simulink model "mcb_bldc_sixstep_f28069mLaunchPad"  (R2023b)
settings: Solver=FixedStepDiscrete  StartTime=0.0  StopTime=2  RelTol=1e-3  EnableMultiTasking=on
InitFcn:
  | mcb_bldc_sixstep_f28069mLaunchPad_data;
values from neighbouring files (symbols this model uses):
  bldc = mcb_SetPMSMMotorParameters('D60MR6430')    [mcb_bldc_sixstep_f28069mLaunchPad_data.m]
  inverter = mcb_SetInverterParameters('SBLMB500')    [mcb_bldc_sixstep_f28069mLaunchPad_data.m]
  PI_params = mcb_SetControllerParameters(bldc,inverter,PU_System,T_pwm,2*Ts,Ts_speed)    [mcb_bldc_sixstep_f28069mLaunchPad_data.m]
  PWM_frequency = 20e3    (= 20000)    [mcb_bldc_sixstep_f28069mLaunchPad_data.m]
  target = mcb_SetProcessorDetails('F28069M',PWM_frequency)    [mcb_bldc_sixstep_f28069mLaunchPad_data.m]
  Ts = 0.03    [dataMonitoringArr.m]    (also in mcb_bldc_sixstep_f28069mLaunchPad_data.m = 5e-05)
  Ts_motor = T_pwm/2    (= 2.5e-05)    [mcb_bldc_sixstep_f28069mLaunchPad_data.m]
  Ts_motor_simscape = T_pwm/100    (= 5e-07)    [mcb_bldc_sixstep_f28069mLaunchPad_data.m]
  Ts_simulink = T_pwm/2    (= 2.5e-05)    [mcb_bldc_sixstep_f28069mLaunchPad_data.m]
  Ts_speed = 10*Ts    (= 0.0005)    [mcb_bldc_sixstep_f28069mLaunchPad_data.m]
undefined symbols (not defined in the file or in its folder): Down, GPTRIP1SEL, GPTRIP2SEL, TZ1, TZ2, Up
libraries: nesl_utility x14, simulink x9, fl_lib x9, c2802xlib x7, mcbcontrolslib x6, c280xlib x6, mcbpositiondecoderlib x5, c2806xlib x5, ee_lib x5, slpidlib x2, svdschedulerlib x2
(part 1 of 3)
settings Model: SILPILSystemUnderTest=refmodels  ExtModeTrigDuration=8  VariantFading=off  Creator=The MathWorks, Inc.  LastModifiedBy=Tefilus
settings SolverCC: AlgebraicLoopSolver=TrustRegion  AutoInsertRateTranBlk=on
settings DataIOCC: LimitDataPoints=on  SaveFormat=Array  SaveOutput=off  SaveTime=off  ReturnWorkspaceOutputs=off
settings OptimizationCC: DefaultParameterBehavior=Inlined  DefaultUnderspecifiedDataType=single  OptimizeBlockIOStorage=off  BufferReuse=off  ReuseModelBlockBuffer=off  GlobalBufferReuse=off  ExpressionFolding=off  ExpressionDepthLimit=2147483647  LocalBlockOutputs=off  InitFltsAndDblsToZero=on  NoFixptDivByZeroProtection=on  EfficientFloat2IntCast=on  EfficientMapNaN2IntZero=off  LifeSpan=inf  MaxStackSize=1024  OptimizeDataStoreBuffers=off  BusAssignmentInplaceUpdate=off  DenormalBehavior=FlushToZero  EfficientTunableParamExpr=on
settings DebuggingCC: AlgebraicLoopMsg=error  ArtificialAlgebraicLoopMsg=error  CheckSSInitialOutputMsg=off  MergeDetectMultiDrivingBlocksExec=none  SolverPrmCheckMsg=warning  InheritedTsInSrcMsg=none  MultiTaskDSMMsg=none  MultiTaskCondExecSysMsg=none  TasksWithSamePriorityMsg=none  SigSpecEnsureSampleTimeMsg=none  ParameterPrecisionLossMsg=none  ParameterTunabilityLossMsg=error  FcnCallInpInsideContextMsg=warning  UnconnectedInputMsg=warning  UnconnectedOutputMsg=warning  UnconnectedLineMsg=warning  AllowSymbolicDim=off  StateNameClashWarn=warning  SFUnexpectedBacktrackingDiag=warning  SFNoUnconditionalDefaultTransitionDiag=warning  SFExecutionAtInitializationDiag=none  ArithmeticOperatorsInVariantConditions=warning
settings HardwareCC: ProdBitPerChar=16  ProdBitPerInt=16  ProdBitPerPointer=32  ProdBitPerSizeT=32  ProdBitPerPtrDiffT=32  ProdLargestAtomicInteger=Integer  ProdLargestAtomicFloat=None  ProdWordSize=16  ProdLongLongMode=on  ProdHWDeviceType=Texas Instruments->C2000  TargetBitPerChar=16  TargetBitPerInt=16  TargetLargestAtomicInteger=Integer  TargetLongLongMode=on  TargetIntDivRoundTo=Zero  TargetEndianess=LittleEndian  TargetWordSize=16  TargetHWDeviceType=Texas Instruments->C2000  ProdEqTarget=off
settings ModelReferenceCC: EnableRefExpFcnMdlSchedulingChecks=on  PropagateSignalLabelsOutOfModel=off
settings SFSimCC: SimUseLocalCustomCode=off  MATLABDynamicMemAlloc=off
settings RTWCC: Description=Embedded Coder  SystemTargetFile=ert.tlc  HardwareBoard=TI Piccolo F28069M LaunchPad  TemplateMakefile=ert_default_tmf  PostCodeGenCommand=; codertarget.postCodeGenHookCommand(h)  GenerateReport=on  RTWUseLocalCustomCode=off  Toolchain=Texas Instruments Code Composer Studio (C2000)  IncludeHyperlinkInReport=on  GenerateTraceInfo=on  GenerateTraceReport=on  GenerateTraceReportSl=on  GenerateTraceReportSf=on  GenerateTraceReportEml=on  DLArmComputeVersion=19.05
settings CodeAppCC: IgnoreCustomStorageClasses=off  CustomSymbolStrType=$N$R$M  StateflowObjectComments=on  InternalIdentifier=Classic
settings ERTTargetCC: TargetFcnLib=ansi_tfl_tmw_new.mat  CodeReplacementLibrary=TI C28x  MultiwordLength=2048  ParMdlRefBuildCompliant=off  CompOptLevelCompliant=off  ConcurrentExecutionCompliant=off  CPPClassGenCompliant=off  ExtModeStaticAllocSize=2000  ExtModeMexFile=TIC2000ExternalModeOpen  ExtModeIntrfLevel=Level2 - Open  ConvertIfToSwitch=off  SuppressUnreachableDefaultCases=off  MemSecPackage=tic2000demospkg
settings ConfigComp: CovMetricSettings=dw  CovSaveCumulativeToWorkspaceVar=on  CovSaveSingleToWorkspaceVar=on  CovExternalEMLEnable=off  CovSFcnEnable=off

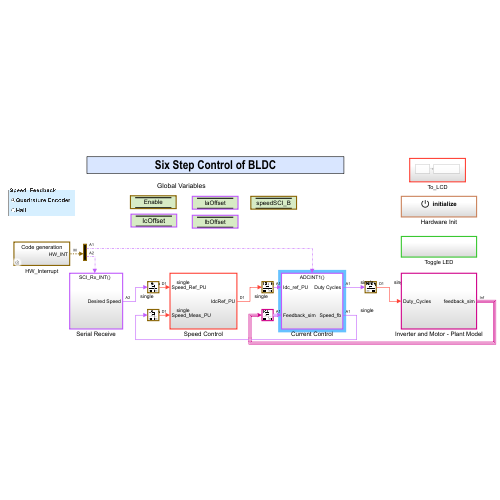
[thumbnail: Simulink's stored preview of the top-level diagram]
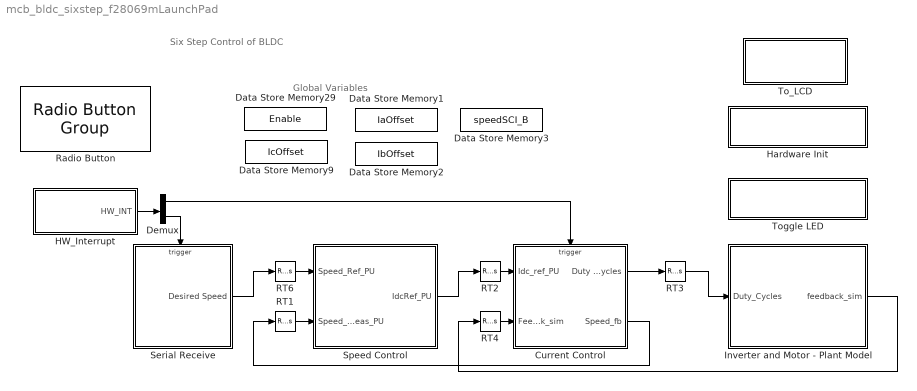
== system mcb_bldc_sixstep_f28069mLaunchPad ==
  note: Six Step Control of BLDC
  note: Global Variables
  Current Control : Subsystem
      settings: RTWSystemCode=Nonreusable function
  Data Store Memory1 : DataStoreMemory  DataStoreName=IaOffset  InitialValue=inverter.CtSensAOffset  ShowAdditionalParam=off
  Data Store Memory2 : DataStoreMemory  DataStoreName=IbOffset  InitialValue=inverter.CtSensBOffset  ShowAdditionalParam=off
  Data Store Memory29 : DataStoreMemory  DataStoreName=Enable  ShowAdditionalParam=off  OutDataTypeStr=boolean
  Data Store Memory3 : DataStoreMemory  DataStoreName=speedSCI_B  InitialValue=inverter.CtSensAOffset  ShowAdditionalParam=off
  Data Store Memory9 : DataStoreMemory  DataStoreName=IcOffset  InitialValue=inverter.CtSensBOffset  ShowAdditionalParam=off
  Demux : Demux  Outputs=2
  HW_Interrupt : Subsystem  Variant=on  VariantControlMode=sim codegen switching
  Hardware Init : Subsystem  TreatAsAtomicUnit=on
  Inverter and Motor - Plant Model : Subsystem
  RT1 : RateTransition  Deterministic=off  OutPortSampleTime=Ts_speed
  RT{2..4,6} (4 alike) : RateTransition  Deterministic=off
  Radio Button : RadioButtonGroup  LabelPosition=Hide  SelectedLabel=Quadrature Encoder  ButtonGroupName=Speed_Feedback
      settings: Values={{'Quadrature Encoder', 'Hall'}, [0 1]}
  Serial Receive : Subsystem  SystemSampleTime=1e-3
  Speed Control : Subsystem  TreatAsAtomicUnit=on  SystemSampleTime=Ts_speed
  To_LCD : Subsystem  TreatAsAtomicUnit=on  SystemSampleTime=Ts_speed
      settings: RTWFcnNameOpts=Use subsystem name  RTWFileNameOpts=Use subsystem name
  Toggle LED : Subsystem
  wires:
  RT3/1 -> Inverter and Motor - Plant Model/1(Duty_Cycles)
  Inverter and Motor - Plant Model/1(feedback_sim) -> RT4/1
  Demux/1 -> Current Control/Trigger
  RT6/1 -> Speed Control/1(Speed_Ref_PU)
  RT1/1 -> Speed Control/2(Speed_Meas_PU)
  Speed Control/1(IdcRef_PU) -> RT2/1
  Demux/2 -> Serial Receive/Trigger
  Current Control/1(Duty Cycles) -> RT3/1
  HW_Interrupt/1(HW_INT) -> Demux/1
  Current Control/2(Speed_fb) -> RT1/1
  RT4/1 -> Current Control/2(Feedback_sim)
  Serial Receive/1(Desired Speed) -> RT6/1
  RT2/1 -> Current Control/1(Idc_ref_PU)

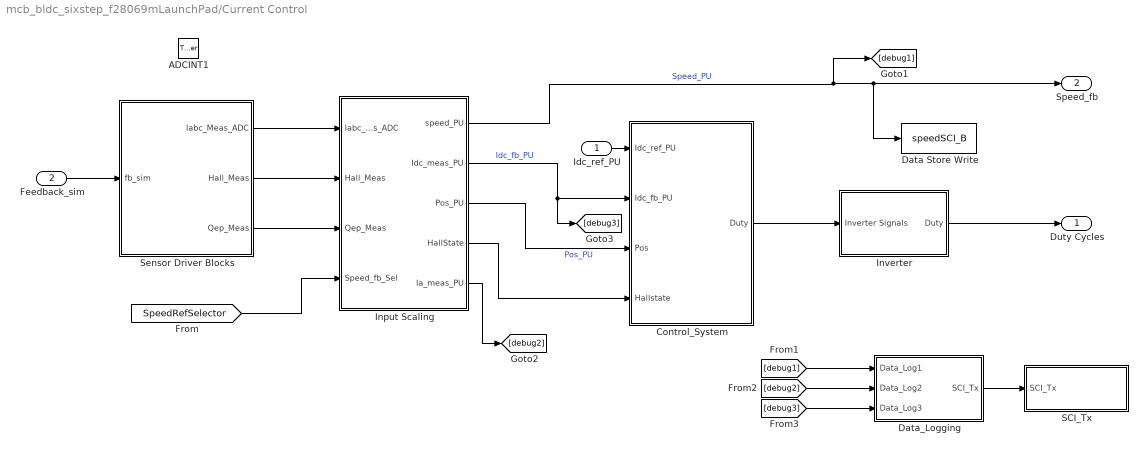
== system mcb_bldc_sixstep_f28069mLaunchPad/Current Control ==
  Idc_ref_PU : Inport
  Feedback_sim : Inport  Port=2
  ADCINT1 : TriggerPort  TriggerType=function-call  VariantControl=Variant  PortDimensions=1
  Control_System : Subsystem
  Data Store Write : DataStoreWrite  DataStoreName=speedSCI_B  IndexOptions=Index vector (dialog)  Indices=1  OutputSizes=1
  Data_Logging : Subsystem
  Input Scaling : Subsystem
  Inverter : Subsystem  Variant=on  VariantControlMode=sim codegen switching
  SCI_Tx : Subsystem  Variant=on  VariantControlMode=sim codegen switching
  Sensor Driver Blocks : Subsystem  Variant=on  VariantControlMode=sim codegen switching
  Duty Cycles : Outport  InitialOutput=0  VectorParamsAs1DForOutWhenUnconnected=off
  Speed_fb : Outport  Port=2  InitialOutput=0  VectorParamsAs1DForOutWhenUnconnected=off
  wires:
  [debug1] -> Data_Logging/1(Data_Log1)
  [debug2] -> Data_Logging/2(Data_Log2)
  Inverter/1(Duty) -> Duty Cycles/1
  Data_Logging/1(SCI_Tx) -> SCI_Tx/1(SCI_Tx)
  [SpeedRefSelector] -> Input Scaling/4(Speed_fb_Sel)
  Sensor Driver Blocks/1(Iabc_Meas_ADC) -> Input Scaling/1(Iabc_meas_ADC)
  Feedback_sim/1 -> Sensor Driver Blocks/1(fb_sim)
  Idc_ref_PU/1 -> Control_System/1(Idc_ref_PU)
  Input Scaling/2(Idc_meas_PU) -> [debug3], Control_System/2(Idc_fb_PU)  "Idc_fb_PU"
  Input Scaling/3(Pos_PU) -> Control_System/3(Pos)  "Pos_PU"
  Input Scaling/4(HallState) -> Control_System/4(Hallstate)
  Input Scaling/1(speed_PU) -> [debug1], Data Store Write/1, Speed_fb/1  "Speed_PU"
  Sensor Driver Blocks/2(Hall_Meas) -> Input Scaling/2(Hall_Meas)
  Sensor Driver Blocks/3(Qep_Meas) -> Input Scaling/3(Qep_Meas)
  Control_System/1(Duty) -> Inverter/1(Inverter Signals)
  Input Scaling/5(Ia_meas_PU) -> [debug2]
  [debug3] -> Data_Logging/3(Data_Log3)

== system mcb_bldc_sixstep_f28069mLaunchPad/HW_Interrupt ==
  Code generation : Subsystem  VariantControl=(codegen)
  Simulation : Subsystem  VariantControl=(sim)
  HW_INT : Outport  OutputFunctionCall=on

== system mcb_bldc_sixstep_f28069mLaunchPad/Hardware Init ==
  6PWM_Mode : Constant  Priority=1000  Value=0x3A16  OutDataTypeStr=uint16  SampleTime=-1
  ADC_Gain_Setting : Constant  Priority=1000  Value=inverter.SPI_Gain_Setting  OutDataTypeStr=uint16  SampleTime=-1
  Event Listener : EventListener  DisableCoverage=on  EventName=reset
  Mux : Mux  Inputs=2
  Variant Subsystem : Subsystem  Variant=on  VariantControlMode=sim codegen switching
  wires:
  6PWM_Mode/1 -> Mux/1
  ADC_Gain_Setting/1 -> Mux/2
  Mux/1 -> Variant Subsystem/1(In1)

== system mcb_bldc_sixstep_f28069mLaunchPad/Inverter and Motor - Plant Model ==
  Duty_Cycles : Inport
  Codegeneration : Subsystem
  Simulation : Subsystem
  Variant Sink : VariantSink  VariantControlMode=sim codegen switching
  Variant Source : VariantSource  VariantControlMode=sim codegen switching
  feedback_sim : Outport  VectorParamsAs1DForOutWhenUnconnected=off
  wires:
  Codegeneration/1(fb_codegen) -> Variant Source/1
  Variant Sink/1 -> Codegeneration/1(Duty_Cycles)
  Variant Source/1 -> feedback_sim/1
  Duty_Cycles/1 -> Variant Sink/1
  Variant Sink/2 -> Simulation/1(Duty_Cycles)
  Simulation/1(fb_sim) -> Variant Source/2

== system mcb_bldc_sixstep_f28069mLaunchPad/Serial Receive ==
  SCI_Rx_INT : TriggerPort  TriggerType=function-call  VariantControl=Variant
  Data Store Write : DataStoreWrite  DataStoreName=Enable  IndexOptions=Index vector (dialog)  Indices=1  OutputSizes=1
  Data Type Conversion1 : DataTypeConversion  OutDataTypeStr=dataType  RndMeth=Simplest  SaturateOnIntegerOverflow=off
  Data Type Conversion3 : DataTypeConversion  OutDataTypeStr=boolean  RndMeth=Simplest  SaturateOnIntegerOverflow=off
  Data_Conditioning : Subsystem
  Demux : Demux  Outputs=2
  SCI_Rx : Subsystem  Variant=on  VariantControlMode=sim codegen switching
  Desired Speed : Outport  VectorParamsAs1DForOutWhenUnconnected=off
  wires:
  SCI_Rx/1(Data) -> Data_Conditioning/1(In1)
  Data Type Conversion1/1 -> Desired Speed/1
  Demux/2 -> Data Type Conversion3/1
  Data_Conditioning/1(Out1) -> Demux/1
  Demux/1 -> Data Type Conversion1/1
  Data Type Conversion3/1 -> Data Store Write/1

== system mcb_bldc_sixstep_f28069mLaunchPad/Speed Control ==
  Speed_Ref_PU : Inport
  Speed_Meas_PU : Inport  Port=2
  PI_Controller_Speed : Subsystem
  Scope : Scope  NumInputPorts=2
  Speed_Ref_Selector : Subsystem
  IdcRef_PU : Outport  VectorParamsAs1DForOutWhenUnconnected=off
  wires:
  Speed_Meas_PU/1 -> Scope/2, PI_Controller_Speed/2(N_fb), Speed_Ref_Selector/2(Speed_Ref_Open)  "Speed_fb"
  Speed_Ref_PU/1 -> Speed_Ref_Selector/1(Speed_Ref_In)  "SpeedRef"
  Speed_Ref_Selector/1(Speed_Ref_PU) -> Scope/1, PI_Controller_Speed/1(N_ref)  "Speed_Ref"
  PI_Controller_Speed/1(Idc_ref) -> IdcRef_PU/1

== system mcb_bldc_sixstep_f28069mLaunchPad/To_LCD ==
  Data_Logging : Subsystem
  SCI_Tx_codegen : Subsystem  TreatAsAtomicUnit=on
  wires:
  Data_Logging/1(SCI_Tx) -> SCI_Tx_codegen/1(SCI_Tx)

== system mcb_bldc_sixstep_f28069mLaunchPad/Toggle LED ==
  Constant : Constant  SampleTime=0.5
  Digital Output1 : c2806xlib/Digital Output  GPIO_Number=GPIO32~GPIO39  GPIO_Bit0=off  GPIO_BIT0_Toggle=off  GPIO_Bit1=off  GPIO_BIT1_Toggle=off  GPIO_Bit2=off  GPIO_BIT2_Toggle=off  GPIO_Bit3=off  GPIO_BIT3_Toggle=off  GPIO_Bit4=off  GPIO_BIT4_Toggle=off  GPIO_Bit5=off  GPIO_BIT5_Toggle=off  GPIO_Bit6=off  GPIO_BIT6_Toggle=off  GPIO_Bit7=on  GPIO_BIT7_Toggle=on
  wires:
  Constant/1 -> Digital Output1/1

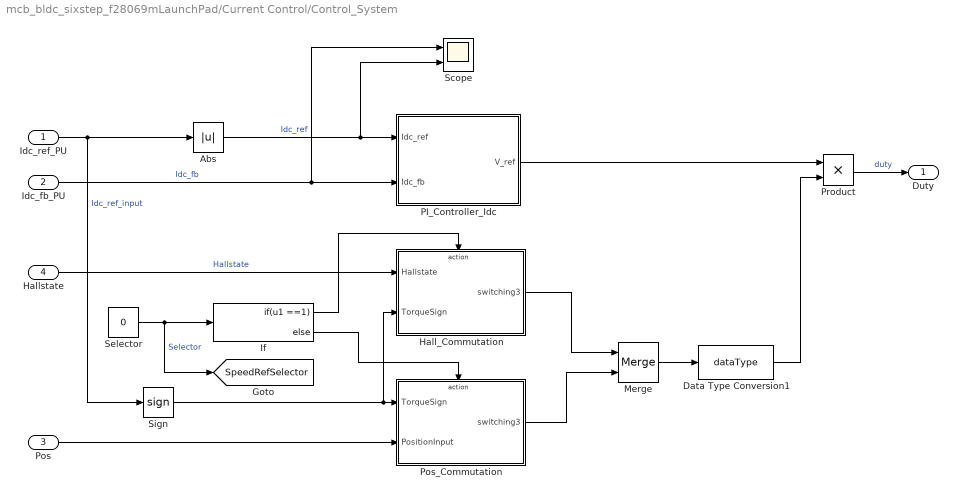
== system mcb_bldc_sixstep_f28069mLaunchPad/Current Control/Control_System ==
  Idc_ref_PU : Inport
  Idc_fb_PU : Inport  Port=2
  Pos : Inport  Port=3
  Hallstate : Inport  Port=4
  Abs : Abs  SaturateOnIntegerOverflow=off
  Data Type Conversion1 : DataTypeConversion  OutDataTypeStr=dataType  RndMeth=Simplest  SaturateOnIntegerOverflow=off
  Hall_Commutation : Subsystem
  If : If  IfExpression=u1 ==1
  Merge : Merge
  PI_Controller_Idc : Subsystem
  Pos_Commutation : Subsystem
  Product : Product  RndMeth=Simplest  OutDataTypeStr=Inherit: Same as first input
  Scope : Scope  NumInputPorts=2
  Selector : Constant  Value=0  OutDataTypeStr=uint16  SampleTime=-1
  Sign : Signum
  Duty : Outport  VectorParamsAs1DForOutWhenUnconnected=off
  tag scope: SpeedRefSelector=global
  wires:
  Hallstate/1 -> Hall_Commutation/1(Hallstate)  "Hallstate"
  Pos/1 -> Pos_Commutation/2(PositionInput)
  If/1 -> Hall_Commutation/Action
  If/2 -> Pos_Commutation/Action
  Pos_Commutation/1(switching3) -> Merge/2
  Hall_Commutation/1(switching3) -> Merge/1
  Merge/1 -> Data Type Conversion1/1
  Idc_fb_PU/1 -> Scope/1, PI_Controller_Idc/2(Idc_fb)  "Idc_fb"
  Abs/1 -> Scope/2, PI_Controller_Idc/1(Idc_ref)  "Idc_ref"
  Idc_ref_PU/1 -> Sign/1, Abs/1  "Idc_ref_input"
  Product/1 -> Duty/1  "duty"
  Selector/1 -> [SpeedRefSelector], If/1  "Selector"
  Sign/1 -> Hall_Commutation/2(TorqueSign), Pos_Commutation/1(TorqueSign)
  Data Type Conversion1/1 -> Product/2
  PI_Controller_Idc/1(V_ref) -> Product/1

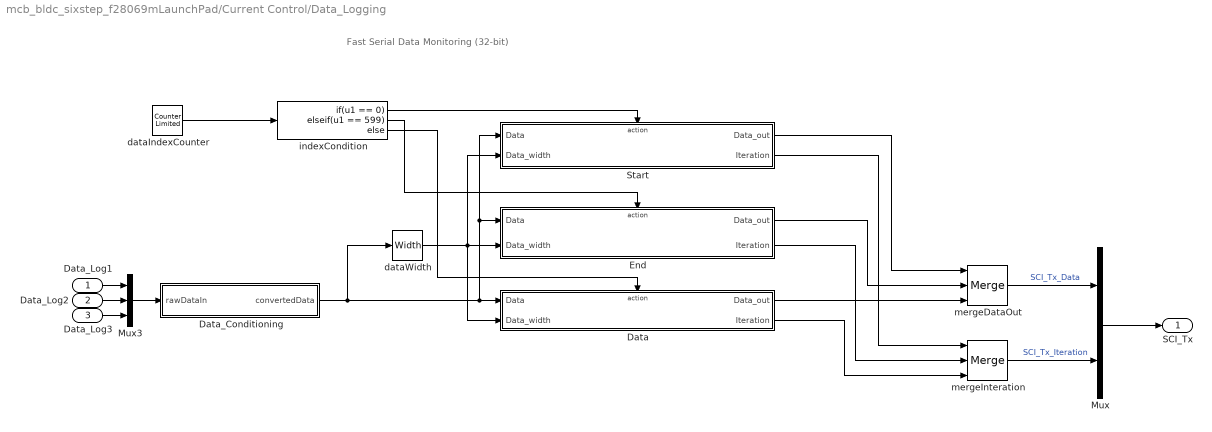
== system mcb_bldc_sixstep_f28069mLaunchPad/Current Control/Data_Logging ==
  note: Fast Serial Data Monitoring (32-bit)
  Data_Log1 : Inport
  Data_Log2 : Inport  Port=2
  Data_Log3 : Inport  Port=3
  Data : Subsystem  TreatAsAtomicUnit=on
  Data_Conditioning : Subsystem
  End : Subsystem  TreatAsAtomicUnit=on
  Mux : Mux  Inputs=2
  Mux3 : Mux  Inputs=3
  Start : Subsystem  TreatAsAtomicUnit=on
  dataIndexCounter : simulink/Sources/Counter Limited  uplimit=600  tsamp=-1
  dataWidth : Width  OutDataTypeMode=All ports same datatype  DataType=uint16
  indexCondition : If  IfExpression=u1 == 0  ElseIfExpressions=u1 == 599
  mergeDataOut : Merge  Inputs=3
  mergeInteration : Merge  Inputs=3
  SCI_Tx : Outport
  wires:
  indexCondition/3 -> Data/Action
  Data/1(Data_out) -> mergeDataOut/3
  dataWidth/1 -> Start/2(Data_width), Data/2(Data_width), End/2(Data_width)
  mergeDataOut/1 -> Mux/1  "SCI_Tx_Data"
  dataIndexCounter/1 -> indexCondition/1
  Start/2(Iteration) -> mergeInteration/1
  Start/1(Data_out) -> mergeDataOut/1
  indexCondition/2 -> End/Action
  mergeInteration/1 -> Mux/2  "SCI_Tx_Iteration"
  indexCondition/1 -> Start/Action
  End/1(Data_out) -> mergeDataOut/2
  End/2(Iteration) -> mergeInteration/2
  Data/2(Iteration) -> mergeInteration/3
  Data_Log1/1 -> Mux3/1
  Data_Conditioning/1(convertedData) -> dataWidth/1, Start/1(Data), End/1(Data), Data/1(Data)
  Mux/1 -> SCI_Tx/1
  Mux3/1 -> Data_Conditioning/1(rawDataIn)
  Data_Log2/1 -> Mux3/2
  Data_Log3/1 -> Mux3/3

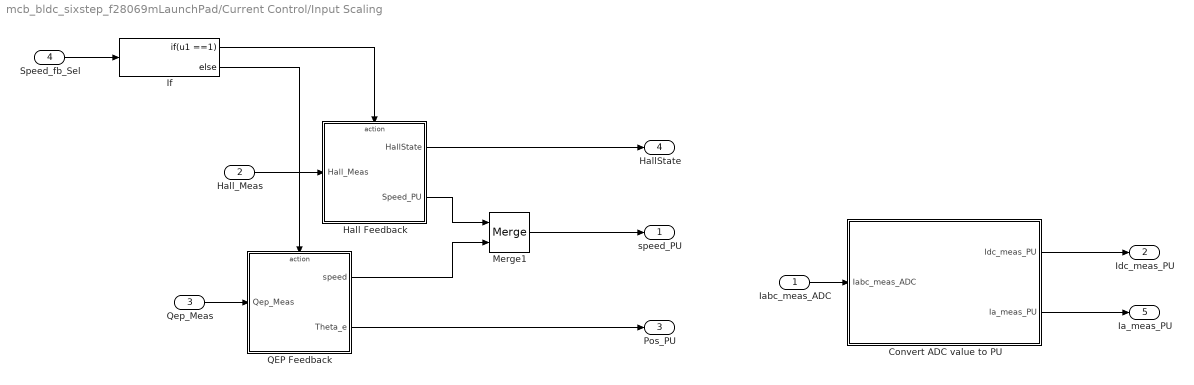
== system mcb_bldc_sixstep_f28069mLaunchPad/Current Control/Input Scaling ==
  Iabc_meas_ADC : Inport
  Hall_Meas : Inport  Port=2
  Qep_Meas : Inport  Port=3
  Speed_fb_Sel : Inport  Port=4
  Convert ADC value to PU : Subsystem
  Hall Feedback : Subsystem  TreatAsAtomicUnit=on
  If : If  IfExpression=u1 ==1
  Merge1 : Merge
  QEP Feedback : Subsystem  TreatAsAtomicUnit=on
  speed_PU : Outport  InitialOutput=0  VectorParamsAs1DForOutWhenUnconnected=off
  Idc_meas_PU : Outport  Port=2  VectorParamsAs1DForOutWhenUnconnected=off
  Pos_PU : Outport  Port=3  InitialOutput=0  VectorParamsAs1DForOutWhenUnconnected=off
  HallState : Outport  Port=4  InitialOutput=0  VectorParamsAs1DForOutWhenUnconnected=off
  Ia_meas_PU : Outport  Port=5  VectorParamsAs1DForOutWhenUnconnected=off
  wires:
  If/2 -> QEP Feedback/Action
  Convert ADC value to PU/2(Ia_meas_PU) -> Ia_meas_PU/1
  Convert ADC value to PU/1(Idc_meas_PU) -> Idc_meas_PU/1
  QEP Feedback/1(speed) -> Merge1/2
  Hall Feedback/2(Speed_PU) -> Merge1/1
  Iabc_meas_ADC/1 -> Convert ADC value to PU/1(Iabc_meas_ADC)
  QEP Feedback/2(Theta_e) -> Pos_PU/1
  Merge1/1 -> speed_PU/1
  Speed_fb_Sel/1 -> If/1
  Hall_Meas/1 -> Hall Feedback/1(Hall_Meas)
  Qep_Meas/1 -> QEP Feedback/1(Qep_Meas)
  If/1 -> Hall Feedback/Action
  Hall Feedback/1(HallState) -> HallState/1

== system mcb_bldc_sixstep_f28069mLaunchPad/Current Control/Inverter ==
  Inverter Signals : Inport
  " Code Generation" : Subsystem  VariantControl=(codegen)
  Simulation : Subsystem  VariantControl=(sim)
  Duty : Outport  VectorParamsAs1DForOutWhenUnconnected=off

== system mcb_bldc_sixstep_f28069mLaunchPad/Current Control/SCI_Tx ==
  SCI_Tx : Inport
  SCI_Tx_codegen : Subsystem  VariantControl=(codegen)
  Simulation : Subsystem  VariantControl=(sim)

== system mcb_bldc_sixstep_f28069mLaunchPad/Current Control/Sensor Driver Blocks ==
  fb_sim : Inport
  Sensor Driver Blocks (codegen) : Subsystem  VariantControl=(codegen)
  Sensor Driver Blocks (sim) : Subsystem  VariantControl=(sim)
  Iabc_Meas_ADC : Outport
  Hall_Meas : Outport  Port=2
  Qep_Meas : Outport  Port=3

== system mcb_bldc_sixstep_f28069mLaunchPad/HW_Interrupt/Code generation ==
  HWI_ADCINT1 : svdschedulerlib/Hardware Interrupt v2  ISRGroup=ADC - Analog to Digital Converter  ISRName=ADCA1_INT  ISRNumber=32  NumEventsToServe=1  EventsList={'on','EOC event','1';'off','Overflow event','2';'off','Custom event','3'}  SelectedEvents={'event1'}  TaskPriority=30  DisablePreemption=off  ClearInterruptFlagsAtEndOfEvent=on  InterruptDefinitionFile=$(TARGET_ROOT)/registry/interrupts/F2837xS_interrupts.xml  HardwareBoard=F2837x  EnableSimPort=off
      settings: LibrarySourceBlock=c2000lib/Scheduling/Hardware Interrupt
  HWI_SCIRXINTA : svdschedulerlib/Hardware Interrupt v2  ISRGroup=ADC - Analog to Digital Converter  ISRName=ADCA1_INT  ISRNumber=32  NumEventsToServe=1  EventsList={'on','EOC event','1';'off','Overflow event','2';'off','Custom event','3'}  SelectedEvents={'event1'}  TaskPriority=50  DisablePreemption=on  ClearInterruptFlagsAtEndOfEvent=on  InterruptDefinitionFile=$(TARGET_ROOT)/registry/interrupts/F2837xS_interrupts.xml  HardwareBoard=F2837x  EnableSimPort=off
      settings: LibrarySourceBlock=c2000lib/Scheduling/Hardware Interrupt
  Mux : Mux  Inputs=2
  HW_INT : Outport
  wires:
  HWI_SCIRXINTA/1 -> Mux/2
  HWI_ADCINT1/1 -> Mux/1
  Mux/1 -> HW_INT/1

== system mcb_bldc_sixstep_f28069mLaunchPad/HW_Interrupt/Simulation ==
  ADCINT1 : simulink/Ports & Subsystems/Function-Call Generator  sample_time=Ts  numberOfIterations=1  DisallowWideOutput=off
  Mux : Mux  Inputs=2
  SCI_Rx_INT : simulink/Ports & Subsystems/Function-Call Generator  sample_time=0.1  numberOfIterations=1  DisallowWideOutput=off
  HW_INT : Outport
  wires:
  SCI_Rx_INT/1 -> Mux/2
  ADCINT1/1 -> Mux/1
  Mux/1 -> HW_INT/1

== system mcb_bldc_sixstep_f28069mLaunchPad/Hardware Init/Variant Subsystem ==
  In1 : Inport
  Code Generation : Subsystem  VariantControl=(codegen)
  Simulation : Subsystem  VariantControl=(sim)

== system mcb_bldc_sixstep_f28069mLaunchPad/Inverter and Motor - Plant Model/Codegeneration ==
  Duty_Cycles : Inport
  Bus Creator : BusCreator  Inputs=3
  Ground : Ground
  Terminator : Terminator
  fb_codegen : Outport  VectorParamsAs1DForOutWhenUnconnected=off
  wires:
  Duty_Cycles/1 -> Terminator/1
  Bus Creator/1 -> fb_codegen/1
  Ground/1 -> Bus Creator/3, Bus Creator/2, Bus Creator/1

== system mcb_bldc_sixstep_f28069mLaunchPad/Inverter and Motor - Plant Model/Simulation ==
  Duty_Cycles : Inport
  Bus Creator : BusCreator  Inputs=3
  Inverter and Motor : Subsystem  VariantControl=get_param([bdroot '/Plant'],'Value')=='0'
  Load_Profile (Torque) : Subsystem
  RT1 : RateTransition  Deterministic=off  OutPortSampleTime=Ts_simulink
  RT2 : RateTransition  Deterministic=off  OutPortSampleTime=Ts_simulink
  RT3 : RateTransition  Deterministic=off  OutPortSampleTime=Ts_simulink
  Sensor_Measurements : Subsystem
  fb_sim : Outport
  wires:
  RT2/1 -> Sensor_Measurements/3(Hall)
  Sensor_Measurements/2(Pos_mech) -> Bus Creator/2  "Pos_fb"
  RT1/1 -> Sensor_Measurements/2(Pos)
  Bus Creator/1 -> fb_sim/1
  Sensor_Measurements/1(Iabc meas ADC) -> Bus Creator/1  "Iabc_fb"
  Sensor_Measurements/3(HallState) -> Bus Creator/3  "Hall_fb"
  Duty_Cycles/1 -> Inverter and Motor/1(Duty_Cycles)
  Load_Profile (Torque)/1(Load_Trq) -> Inverter and Motor/2(Load)
  Inverter and Motor/1(Iabc) -> RT3/1
  Inverter and Motor/2(Theta) -> RT1/1
  Inverter and Motor/3(Hall) -> RT2/1
  RT3/1 -> Sensor_Measurements/1(Iabc meas)

== system mcb_bldc_sixstep_f28069mLaunchPad/Serial Receive/Data_Conditioning ==
  In1 : Inport
  Data Type Conversion1 : DataTypeConversion  OutDataTypeStr=single  RndMeth=Simplest  SaturateOnIntegerOverflow=off
  Data Type Conversion2 : DataTypeConversion  OutDataTypeStr=fixdt(1,16,12)  ConvertRealWorld=Stored Integer (SI)  RndMeth=Simplest  SaturateOnIntegerOverflow=off
  Out1 : Outport  VectorParamsAs1DForOutWhenUnconnected=off
  wires:
  Data Type Conversion1/1 -> Out1/1
  In1/1 -> Data Type Conversion2/1
  Data Type Conversion2/1 -> Data Type Conversion1/1

== system mcb_bldc_sixstep_f28069mLaunchPad/Serial Receive/SCI_Rx ==
  Code Generation : Subsystem  VariantControl=(codegen)
  Simulation : Subsystem  VariantControl=(sim)
  Data : Outport

== system mcb_bldc_sixstep_f28069mLaunchPad/Speed Control/PI_Controller_Speed ==
  N_ref : Inport
  N_fb : Inport  Port=2
  Data Store Read2 : DataStoreRead  DataStoreName=Enable  IndexOptions=Index vector (dialog)  Indices=1  OutputSizes=1
  Discrete PI Controller with anti-windup & reset : slpidlib/PID Controller  Controller=PI  Form=Parallel  TimeDomain=Discrete-time  UseExternalTs=off  SampleTime=-1  IntegratorMethod=Forward Euler  FilterMethod=Forward Euler  ControllerParametersSource=external  P=1  I=1  UseKiTs=on  D=0  N=100  UseFilter=on  TunerSelectOption=Transfer Function Based (PID Tuner App)  InitialConditionSource=external  InitialConditionForIntegrator=0  InitialConditionForFilter=0  DifferentiatorICPrevScaledInput=0  ExternalReset=level  TrackingMode=off  Kt=1  LimitOutput=on  SatLimitsSource=internal  UpperSaturationLimit=1  LowerSaturationLimit=-1  LinearizeAsGain=on  AntiWindupMode=clamping  Kb=1  LimitIntegrator=off  UpperIntegratorSaturationLimit=inf  LowerIntegratorSaturationLimit=-inf  RndMeth=Simplest  POutMin=[]  POutMax=[]  IOutMin=[]  IOutMax=[]  DOutMin=[]  DOutMax=[]  NOutMin=[]  NOutMax=[]  SumOutMin=[]  SumOutMax=[]  SaturationOutDataTypeStr=Inherit: Inherit via back propagation  SaturationOutMin=[]  SaturationOutMax=[]  PParamMin=[]  PParamMax=[]  IParamMin=[]  IParamMax=[]  DParamMin=[]  DParamMax=[]  NParamMin=[]  NParamMax=[]  KbParamMin=[]  KbParamMax=[]  KtParamMin=[]  KtParamMax=[]  KbOutMin=[]  KbOutMax=[]  KtOutMin=[]  KtOutMax=[]  IntegratorOutMin=[]  IntegratorOutMax=[]  FilterOutMin=[]  FilterOutMax=[]  SumI1OutMin=[]  SumI1OutMax=[]  SumI2OutMin=[]  SumI2OutMax=[]  SumI3OutMin=[]  SumI3OutMax=[]  SumI4OutMin=[]  SumI4OutMax=[]  SumDOutMin=[]  SumDOutMax=[]  DifferentiatorOutMin=[]  DifferentiatorOutMax=[]  FilterDiffOutCoefMin=[]  FilterDiffOutCoefMax=[]  ReciprocalOutMin=[]  ReciprocalOutMax=[]  SumDenOutMin=[]  SumDenOutMax=[]  SumNumOutMin=[]  SumNumOutMax=[]  DivideOutMin=[]  DivideOutMax=[]  UdiffTsProdOutMin=[]  UdiffTsProdOutMax=[]  NTsProdOutMin=[]  NTsProdOutMax=[]  UintegralTsProdOutMin=[]  UintegralTsProdOutMax=[]  UngainTsProdOutMin=[]  UngainTsProdOutMax=[]  ClampingZeroOutDataTypeStr=Inherit: Inherit via back propagation  ClampingZeroOutMin=[]  ClampingZeroOutMax=[]  FilterDenConstantOutDataTypeStr=Inherit: Inherit via back propagation  FilterDenConstantOutMin=[]  FilterDenConstantOutMax=[]  PCopyOutDataTypeStr=Inherit: Inherit via back propagation  PCopyOutMin=[]  PCopyOutMax=[]  NCopyOutDataTypeStr=Inherit: Inherit via back propagation  NCopyOutMin=[]  NCopyOutMax=[]  IntegratorContinuousStateAttributes=''  IntegratorStateMustResolveToSignalObject=off  IntegratorRTWStateStorageClass=Auto  FilterContinuousStateAttributes=''  FilterStateMustResolveToSignalObject=off  FilterRTWStateStorageClass=Auto  ParallelPVariant=ExternalParameters  IdealPVariant=Disabled  IVariant=ExternalParameters  DVariant=Disabled  IntegratorVariant=Discrete  SatVariant=Enabled  AWVariant=DiscClampingParallel  PCopyVariant=Disabled  TRVariant=Disabled  FdbkBlocksVariant=Forward  IdealPFdbkVariant=Disabled  SatFdbkVariant=Disabled  DerivativeFilterVariant=Disabled  NVariant=Disabled  NCopyVariant=Disabled_SignalSpec  FilterICVariant=Disabled  IntegratorICVariant=ExternalICs  ExternalResetVariant=ExternalReset  TRSumVariant=Passthrough  SumFdbkVariant=Disabled  SumVariant=Sum_PI  TsampFilterVariant=InternalTs  TsampNgainVariant=Passthrough  TsampIntegralVariant=Disabled_SignalSpec  ExternalSaturationOutDataTypeStr=Inherit: Same as second input
      settings: LibrarySourceBlock=mcbcontrolslib/PI Controller
  Ki1 : Constant  Value=PI_params.Ki_speed*Ts_speed  OutDataTypeStr=dataType  SampleTime=-1
  Ki2 : Constant  Value=0  OutDataTypeStr=dataType  SampleTime=-1
  Kp1 : Constant  Value=PI_params.Kp_speed  OutDataTypeStr=dataType  SampleTime=-1
  Logical Operator : Logic  Operator=NOT  IconShape=distinctive  AllPortsSameDT=off  OutDataTypeStr=boolean
  Sum : Sum  Inputs=|+-  RndMeth=Round
  Zero_Cancellation : mcbcontrolslib/IIR Filter  VariantControl=Low Pass Filter  VariantSelect=Low-pass  Filter_constant=0.01*(Ts_speed/Ts)  advancedSettings=off  Ts=50e-6  cutOff_freq=353.6777
  Idc_ref : Outport  VectorParamsAs1DForOutWhenUnconnected=off
  wires:
  Discrete PI Controller with anti-windup & reset/1 -> Idc_ref/1
  Ki1/1 -> Discrete PI Controller with anti-windup & reset/3
  Kp1/1 -> Discrete PI Controller with anti-windup & reset/2
  N_fb/1 -> Sum/2
  N_ref/1 -> Zero_Cancellation/1
  Logical Operator/1 -> Discrete PI Controller with anti-windup & reset/4
  Ki2/1 -> Discrete PI Controller with anti-windup & reset/5
  Sum/1 -> Discrete PI Controller with anti-windup & reset/1
  Data Store Read2/1 -> Logical Operator/1
  Zero_Cancellation/1 -> Sum/1

== system mcb_bldc_sixstep_f28069mLaunchPad/Speed Control/Speed_Ref_Selector ==
  Speed_Ref_In : Inport
  Speed_Ref_Open : Inport  Port=2
  Data Store Read1 : DataStoreRead  DataStoreName=Enable  IndexOptions=Index vector (dialog)  Indices=1  OutputSizes=1
  Switch : Switch  Criteria=u2 > Threshold  Threshold=0.5  SaturateOnIntegerOverflow=off  InputSameDT=off
  Speed_Ref_PU : Outport
  wires:
  Switch/1 -> Speed_Ref_PU/1
  Data Store Read1/1 -> Switch/2
  Speed_Ref_Open/1 -> Switch/3
  Speed_Ref_In/1 -> Switch/1

== system mcb_bldc_sixstep_f28069mLaunchPad/To_LCD/Data_Logging ==
  Data : Subsystem  TreatAsAtomicUnit=on
  Data_Conditioning : Subsystem
  End : Subsystem  TreatAsAtomicUnit=on
  Mux : Mux  Inputs=2
  Start : Subsystem  TreatAsAtomicUnit=on
  dataIndexCounter : simulink/Sources/Counter Limited  uplimit=600  tsamp=-1
  dataLogging_Speed : DataStoreRead  DataStoreName=speedSCI_B  IndexOptions=Index vector (dialog)  Indices=1  OutputSizes=1
  dataWidth : Width  OutDataTypeMode=All ports same datatype  DataType=uint16
  indexCondition : If  IfExpression=u1 == 0  ElseIfExpressions=u1 == 599
  mergeDataOut : Merge  Inputs=3
  mergeInteration : Merge  Inputs=3
  SCI_Tx : Outport
  wires:
  indexCondition/3 -> Data/Action
  Data/1(Data_out) -> mergeDataOut/3
  dataWidth/1 -> Start/2(Data_width), Data/2(Data_width), End/2(Data_width)
  mergeDataOut/1 -> Mux/1  "SCI_Tx_Data"
  dataIndexCounter/1 -> indexCondition/1
  Start/2(Iteration) -> mergeInteration/1
  Start/1(Data_out) -> mergeDataOut/1
  indexCondition/2 -> End/Action
  mergeInteration/1 -> Mux/2  "SCI_Tx_Iteration"
  indexCondition/1 -> Start/Action
  End/1(Data_out) -> mergeDataOut/2
  End/2(Iteration) -> mergeInteration/2
  Data/2(Iteration) -> mergeInteration/3
  Data_Conditioning/1(convertedData) -> dataWidth/1, Start/1(Data), End/1(Data), Data/1(Data)
  Mux/1 -> SCI_Tx/1
  dataLogging_Speed/1 -> Data_Conditioning/1(rawDataIn)

== system mcb_bldc_sixstep_f28069mLaunchPad/To_LCD/SCI_Tx_codegen ==
  SCI_Tx : Inport
  Add : Sum  Inputs=+-  OutDataTypeStr=Inherit: Same as first input
  Demux2 : Demux  Outputs=2
  Index Vector : MultiPortSwitch  Inputs=1  SaturateOnIntegerOverflow=off  InputSameDT=off
  SCI Transmit : c280xlib/SCI Transmit  sciModule=B  dataHead=''  dataTail=''  frameSize=1  blockingMode=on  outputStatus=off
  While Iterator : WhileIterator  MaxIters=-1  WhileBlockType=do-while  ShowIterationPort=on  OutputDataType=int16
  wires:
  While Iterator/1 -> Add/2, Index Vector/1
  Demux2/1 -> Index Vector/2
  Index Vector/1 -> SCI Transmit/1
  Add/1 -> While Iterator/1
  Demux2/2 -> Add/1
  SCI_Tx/1 -> Demux2/1

== system mcb_bldc_sixstep_f28069mLaunchPad/Current Control/Control_System/Hall_Commutation ==
  Hallstate : Inport
  TorqueSign : Inport  Port=2
  Action Port : ActionPort  ActionPortLabel=if(u1 ==1)
  Six Step Commutation : mcbcontrolslib/Six Step Commutation  InputType=Hall  PositionUnit=Per unit  CommutationMode=120 deg  SequencePos=bldc.HallSequence  EnableCustomSwitching=off  CommutationSeqPos=hallCommutation  CommutationSeqNeg="[0  1  1  0  0  0;0  1  0  0  1  0;0  0  0  1  1  0;1  0  0  1  0  0;1  0  0  0  0  1;0  0  1  0  0  1;]"
  switching3 : Outport
  wires:
  Hallstate/1 -> Six Step Commutation/1
  Six Step Commutation/1 -> switching3/1  "switching"
  TorqueSign/1 -> Six Step Commutation/2

== system mcb_bldc_sixstep_f28069mLaunchPad/Current Control/Control_System/PI_Controller_Idc ==
  Idc_ref : Inport
  Idc_fb : Inport  Port=2
  Data Store Read1 : DataStoreRead  DataStoreName=Enable  IndexOptions=Index vector (dialog)  Indices=1  OutputSizes=1
  Discrete PI Controller with anti-windup & reset : slpidlib/PID Controller  Controller=PI  Form=Parallel  TimeDomain=Discrete-time  UseExternalTs=off  SampleTime=-1  IntegratorMethod=Forward Euler  FilterMethod=Forward Euler  ControllerParametersSource=external  P=1  I=1  UseKiTs=on  D=0  N=100  UseFilter=on  TunerSelectOption=Transfer Function Based (PID Tuner App)  InitialConditionSource=external  InitialConditionForIntegrator=0  InitialConditionForFilter=0  DifferentiatorICPrevScaledInput=0  ExternalReset=level  TrackingMode=off  Kt=1  LimitOutput=on  SatLimitsSource=internal  UpperSaturationLimit=1  LowerSaturationLimit=0  LinearizeAsGain=on  AntiWindupMode=clamping  Kb=1  LimitIntegrator=off  UpperIntegratorSaturationLimit=inf  LowerIntegratorSaturationLimit=-inf  RndMeth=Simplest  POutMin=[]  POutMax=[]  IOutMin=[]  IOutMax=[]  DOutMin=[]  DOutMax=[]  NOutMin=[]  NOutMax=[]  SumOutMin=[]  SumOutMax=[]  SaturationOutDataTypeStr=Inherit: Inherit via back propagation  SaturationOutMin=[]  SaturationOutMax=[]  PParamMin=[]  PParamMax=[]  IParamMin=[]  IParamMax=[]  DParamMin=[]  DParamMax=[]  NParamMin=[]  NParamMax=[]  KbParamMin=[]  KbParamMax=[]  KtParamMin=[]  KtParamMax=[]  KbOutMin=[]  KbOutMax=[]  KtOutMin=[]  KtOutMax=[]  IntegratorOutMin=[]  IntegratorOutMax=[]  FilterOutMin=[]  FilterOutMax=[]  SumI1OutMin=[]  SumI1OutMax=[]  SumI2OutMin=[]  SumI2OutMax=[]  SumI3OutMin=[]  SumI3OutMax=[]  SumI4OutMin=[]  SumI4OutMax=[]  SumDOutMin=[]  SumDOutMax=[]  DifferentiatorOutMin=[]  DifferentiatorOutMax=[]  FilterDiffOutCoefMin=[]  FilterDiffOutCoefMax=[]  ReciprocalOutMin=[]  ReciprocalOutMax=[]  SumDenOutMin=[]  SumDenOutMax=[]  SumNumOutMin=[]  SumNumOutMax=[]  DivideOutMin=[]  DivideOutMax=[]  UdiffTsProdOutMin=[]  UdiffTsProdOutMax=[]  NTsProdOutMin=[]  NTsProdOutMax=[]  UintegralTsProdOutMin=[]  UintegralTsProdOutMax=[]  UngainTsProdOutMin=[]  UngainTsProdOutMax=[]  ClampingZeroOutDataTypeStr=Inherit: Inherit via back propagation  ClampingZeroOutMin=[]  ClampingZeroOutMax=[]  FilterDenConstantOutDataTypeStr=Inherit: Inherit via back propagation  FilterDenConstantOutMin=[]  FilterDenConstantOutMax=[]  PCopyOutDataTypeStr=Inherit: Inherit via back propagation  PCopyOutMin=[]  PCopyOutMax=[]  NCopyOutDataTypeStr=Inherit: Inherit via back propagation  NCopyOutMin=[]  NCopyOutMax=[]  IntegratorContinuousStateAttributes=''  IntegratorStateMustResolveToSignalObject=off  IntegratorRTWStateStorageClass=Auto  FilterContinuousStateAttributes=''  FilterStateMustResolveToSignalObject=off  FilterRTWStateStorageClass=Auto  ParallelPVariant=ExternalParameters  IdealPVariant=Disabled  IVariant=ExternalParameters  DVariant=Disabled  IntegratorVariant=Discrete  SatVariant=Enabled  AWVariant=DiscClampingParallel  PCopyVariant=Disabled  TRVariant=Disabled  FdbkBlocksVariant=Forward  IdealPFdbkVariant=Disabled  SatFdbkVariant=Disabled  DerivativeFilterVariant=Disabled  NVariant=Disabled  NCopyVariant=Disabled_SignalSpec  FilterICVariant=Disabled  IntegratorICVariant=ExternalICs  ExternalResetVariant=ExternalReset  TRSumVariant=Passthrough  SumFdbkVariant=Disabled  SumVariant=Sum_PI  TsampFilterVariant=InternalTs  TsampNgainVariant=Passthrough  TsampIntegralVariant=Disabled_SignalSpec  ExternalSaturationOutDataTypeStr=Inherit: Same as second input
      settings: LibrarySourceBlock=mcbcontrolslib/PI Controller
  Ki : Constant  Value=PI_params.Ki_i*Ts*0  OutDataTypeStr=dataType  SampleTime=-1
  Kp : Constant  Value=PI_params.Kp_i  OutDataTypeStr=dataType  SampleTime=-1
  Kp1 : Constant  Value=0  OutDataTypeStr=dataType  SampleTime=-1
  Logical Operator : Logic  Operator=NOT  IconShape=distinctive  AllPortsSameDT=off  OutDataTypeStr=boolean
  Sum : Sum  Inputs=|+-  OutDataTypeStr=Inherit: Same as first input
  V_ref : Outport  VectorParamsAs1DForOutWhenUnconnected=off
  wires:
  Discrete PI Controller with anti-windup & reset/1 -> V_ref/1
  Data Store Read1/1 -> Logical Operator/1
  Idc_fb/1 -> Sum/2
  Idc_ref/1 -> Sum/1
  Sum/1 -> Discrete PI Controller with anti-windup & reset/1
  Logical Operator/1 -> Discrete PI Controller with anti-windup & reset/4
  Kp1/1 -> Discrete PI Controller with anti-windup & reset/5
  Kp/1 -> Discrete PI Controller with anti-windup & reset/2
  Ki/1 -> Discrete PI Controller with anti-windup & reset/3

== system mcb_bldc_sixstep_f28069mLaunchPad/Current Control/Control_System/Pos_Commutation ==
  TorqueSign : Inport
  PositionInput : Inport  Port=2
  Action Port : ActionPort  ActionPortLabel=else
  Six Step Commutation : mcbcontrolslib/Six Step Commutation  InputType=Position  PositionUnit=Per unit  CommutationMode=120 deg  SequencePos=[5,4,6,2,3,1]  EnableCustomSwitching=off  CommutationSeqPos=[1 0 0 1 0 0;1 0 0 0 0 1; 0 0 1 0 0 1;0 1 1 0 0 0;0 1 0 0 1 0;0 0 0 1 1 0]  CommutationSeqNeg="[0  1  1  0  0  0;0  1  0  0  1  0;0  0  0  1  1  0;1  0  0  1  0  0;1  0  0  0  0  1;0  0  1  0  0  1;]"
  switching3 : Outport
  wires:
  PositionInput/1 -> Six Step Commutation/1
  TorqueSign/1 -> Six Step Commutation/2
  Six Step Commutation/1 -> switching3/1  "switching"

== system mcb_bldc_sixstep_f28069mLaunchPad/Current Control/Data_Logging/Data ==
  Data : Inport
  Data_width : Inport  Port=2
  Action Port : ActionPort  ActionPortLabel=else
  Mux : Mux  Inputs=2
  Start : Constant  Value=hex2dec('0000')  OutDataTypeStr=uint16
  Data_out : Outport  VectorParamsAs1DForOutWhenUnconnected=off
  Iteration : Outport  Port=2  VectorParamsAs1DForOutWhenUnconnected=off
  wires:
  Start/1 -> Mux/2
  Mux/1 -> Data_out/1
  Data/1 -> Mux/1
  Data_width/1 -> Iteration/1

== system mcb_bldc_sixstep_f28069mLaunchPad/Current Control/Data_Logging/Data_Conditioning ==
  rawDataIn : Inport
  convertTo_sfix16_En12 : DataTypeConversion  OutDataTypeStr=fixdt(1,16,12)  RndMeth=Simplest  SaturateOnIntegerOverflow=off
  convertTo_uint16 : DataTypeConversion  OutDataTypeStr=uint16  ConvertRealWorld=Stored Integer (SI)  SaturateOnIntegerOverflow=off  RndMeth=Floor
  convertedData : Outport  VectorParamsAs1DForOutWhenUnconnected=off
  wires:
  rawDataIn/1 -> convertTo_sfix16_En12/1
  convertTo_uint16/1 -> convertedData/1
  convertTo_sfix16_En12/1 -> convertTo_uint16/1

== system mcb_bldc_sixstep_f28069mLaunchPad/Current Control/Data_Logging/End ==
  Data : Inport
  Data_width : Inport  Port=2
  Action Port : ActionPort  ActionPortLabel=elseif(u1 == 599)
  Bias : Bias  Bias=1  SaturateOnIntegerOverflow=off
  Mux : Mux  Inputs=2
  Start : Constant  Value=hex2dec('4545')  OutDataTypeStr=uint16
  Data_out : Outport  VectorParamsAs1DForOutWhenUnconnected=off
  Iteration : Outport  Port=2  VectorParamsAs1DForOutWhenUnconnected=off
  wires:
  Mux/1 -> Data_out/1
  Data_width/1 -> Bias/1
  Start/1 -> Mux/2
  Bias/1 -> Iteration/1
  Data/1 -> Mux/1

== system mcb_bldc_sixstep_f28069mLaunchPad/Current Control/Data_Logging/Start ==
  Data : Inport
  Data_width : Inport  Port=2
  Action Port : ActionPort  ActionPortLabel=if(u1 == 0)
  Bias : Bias  Bias=1  SaturateOnIntegerOverflow=off
  End : Constant  Value=hex2dec('5353')  OutDataTypeStr=uint16
  Mux : Mux  Inputs=2
  Data_out : Outport  VectorParamsAs1DForOutWhenUnconnected=off
  Iteration : Outport  Port=2  VectorParamsAs1DForOutWhenUnconnected=off
  wires:
  End/1 -> Mux/1
  Mux/1 -> Data_out/1
  Data_width/1 -> Bias/1
  Bias/1 -> Iteration/1
  Data/1 -> Mux/2

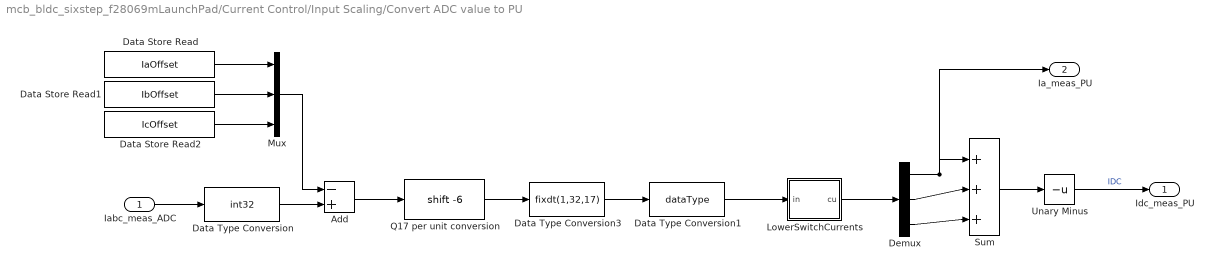
== system mcb_bldc_sixstep_f28069mLaunchPad/Current Control/Input Scaling/Convert ADC value to PU ==
  Iabc_meas_ADC : Inport
  Add : Sum  Inputs=-+
  Data Store Read : DataStoreRead  DataStoreName=IaOffset  IndexOptions=Index vector (dialog)  Indices=1  OutputSizes=1
  Data Store Read1 : DataStoreRead  DataStoreName=IbOffset  IndexOptions=Index vector (dialog)  Indices=1  OutputSizes=1
  Data Store Read2 : DataStoreRead  DataStoreName=IcOffset  IndexOptions=Index vector (dialog)  Indices=1  OutputSizes=1
  Data Type Conversion : DataTypeConversion  OutDataTypeStr=int32  ConvertRealWorld=Stored Integer (SI)  SaturateOnIntegerOverflow=off  RndMeth=Floor
  Data Type Conversion1 : DataTypeConversion  OutDataTypeStr=dataType  SaturateOnIntegerOverflow=off  RndMeth=Floor
  Data Type Conversion3 : DataTypeConversion  OutDataTypeStr=fixdt(1,32,17)  ConvertRealWorld=Stored Integer (SI)  RndMeth=Simplest  SaturateOnIntegerOverflow=off
  Demux : Demux  Outputs=3
  LowerSwitchCurrents : Subsystem
  Mux : Mux  Inputs=3
  Q17 per unit conversion : ArithShift  BitShiftNumber=-6
  Sum : Sum  Inputs=|+++
  Unary Minus : UnaryMinus
  Idc_meas_PU : Outport
  Ia_meas_PU : Outport  Port=2
  wires:
  Data Type Conversion3/1 -> Data Type Conversion1/1
  Q17 per unit conversion/1 -> Data Type Conversion3/1
  Demux/2 -> Sum/2
  Demux/1 -> Ia_meas_PU/1, Sum/1
  Demux/3 -> Sum/3
  Data Type Conversion1/1 -> LowerSwitchCurrents/1(in)
  Data Store Read2/1 -> Mux/3
  Data Store Read1/1 -> Mux/2
  Data Store Read/1 -> Mux/1
  Iabc_meas_ADC/1 -> Data Type Conversion/1
  Data Type Conversion/1 -> Add/2
  Mux/1 -> Add/1
  Add/1 -> Q17 per unit conversion/1
  Unary Minus/1 -> Idc_meas_PU/1  "IDC"
  LowerSwitchCurrents/1(cu) -> Demux/1
  Sum/1 -> Unary Minus/1

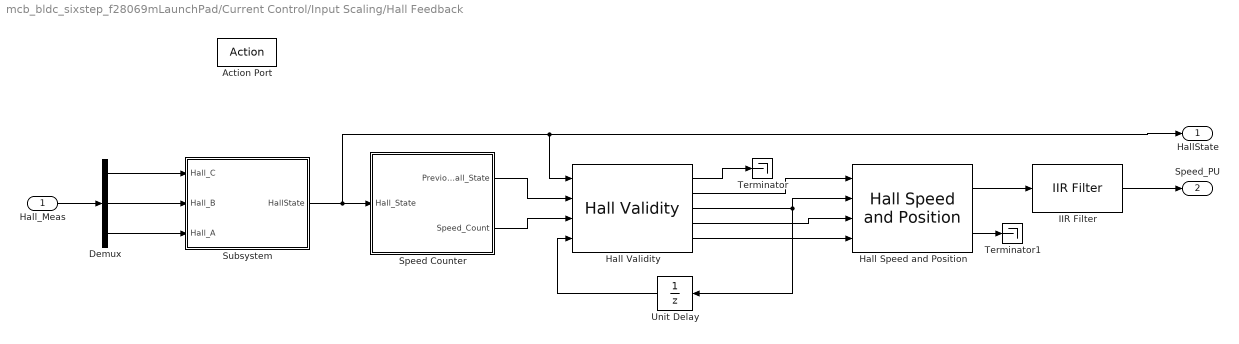
== system mcb_bldc_sixstep_f28069mLaunchPad/Current Control/Input Scaling/Hall Feedback ==
  Hall_Meas : Inport
  Action Port : ActionPort  ActionPortLabel=if(u1 ==1)
  Demux : Demux  Outputs=3
  Hall Speed and Position : mcbpositiondecoderlib/Hall Speed and Position  blkExecutionType=Speed  CounterSize=32 bits  ClkFreq=1/Ts  BlkSampleTime=Ts  PolePairs=bldc.p  MinSpeed=20  HallInterruptConfig=Every 60 Degrees  SpeedUnit=Per unit  PerUnitSpeed=PU_System.N_base  SpeedDataType=dataType  hallSequence=ABC  Sequence=[5,4,6,2,3,1]  EnableSecondOrder=1st Order  PositionUnit=Radians  PositionDataType=single
  Hall Validity : mcbpositiondecoderlib/Hall Validity  hallSequence=Custom sequence  sequence=bldc.HallSequence  CounterSize=32 bits
  IIR Filter : mcbcontrolslib/IIR Filter  VariantControl=Low Pass Filter  VariantSelect=Low-pass  Filter_constant=0.01  advancedSettings=off  Ts=50e-6  cutOff_freq=32.1525
  Speed Counter : Subsystem
  Subsystem : Subsystem
  Terminator : Terminator
  Terminator1 : Terminator
  Unit Delay : UnitDelay  InitialCondition=1  SampleTime=-1  HasFrameUpgradeWarning=on
  HallState : Outport  InitialOutput=0  VectorParamsAs1DForOutWhenUnconnected=off
  Speed_PU : Outport  Port=2  InitialOutput=0  VectorParamsAs1DForOutWhenUnconnected=off
  wires:
  Hall Speed and Position/1 -> IIR Filter/1
  Hall Speed and Position/2 -> Terminator1/1
  Hall Validity/2 -> Hall Speed and Position/1
  Hall Validity/3 -> Hall Speed and Position/2, Unit Delay/1
  Hall Validity/4 -> Hall Speed and Position/3
  Hall Validity/5 -> Hall Speed and Position/4
  Speed Counter/2(Speed_Count) -> Hall Validity/3
  Speed Counter/1(Previous_Hall_State) -> Hall Validity/2
  Subsystem/1(HallState) -> HallState/1, Hall Validity/1, Speed Counter/1(Hall_State)
  Unit Delay/1 -> Hall Validity/4
  Hall Validity/1 -> Terminator/1
  Demux/1 -> Subsystem/1(Hall_C)
  Demux/2 -> Subsystem/2(Hall_B)
  Demux/3 -> Subsystem/3(Hall_A)
  Hall_Meas/1 -> Demux/1
  IIR Filter/1 -> Speed_PU/1

== system mcb_bldc_sixstep_f28069mLaunchPad/Current Control/Input Scaling/QEP Feedback ==
  Qep_Meas : Inport
  Action Port : ActionPort  ActionPortLabel=else
  " Calculate Position and Speed" : Subsystem
  Demux : Demux  Outputs=2
  IndexOffset : Constant  Value=bldc.PositionOffset  OutDataTypeStr=dataType  SampleTime=-1
  speed : Outport
  Theta_e : Outport  Port=2
  wires:
  Demux/1 -> " Calculate Position and Speed"/1(QEP_Position_Count)
  IndexOffset/1 -> " Calculate Position and Speed"/3(Offset)
  Demux/2 -> " Calculate Position and Speed"/2(QEP_Index_Latch)
  " Calculate Position and Speed"/1(Theta_e) -> Theta_e/1
  Qep_Meas/1 -> Demux/1
  " Calculate Position and Speed"/2(speed) -> speed/1
